simulink model "cart_model"  (R2015b)
settings: Solver=VariableStepAuto  StartTime=0.0  StopTime=20  RelTol=1e-3
InitFcn:
  | [g,m1,T1,f_1s,f_1k,m2,l,f_2k,M_sp,f_1k_lin,f_2k_lin,k1,k2] =...
  |     set_system_parameters()
values from neighbouring files (symbols this model uses):
  f_1k = f_1s * 0.9    (= 0.143348623853)    [set_system_parameters.m]
  f_1k_lin = 8    [set_system_parameters.m]
  f_1s = T1 / (m1 * g)    (= 0.159276248726)    [set_system_parameters.m]
  f_2k = 0.0062586    [set_system_parameters.m]
  f_2k_lin = 0.01    [set_system_parameters.m]
  g = 9.81    [set_system_parameters.m]
  k1 = -200    [set_system_parameters.m]
  k2 = -5    [set_system_parameters.m]
  l = 2/3 * l_physical    (= 0.466666666667)    [set_system_parameters.m]
  m1 = 1.6    [set_system_parameters.m]
  m2 = 55/1000    (= 0.055)    [set_system_parameters.m]
  M_sp = 0.0065    [set_system_parameters.m]
undefined symbols (not defined in the file or in its folder): sgn, zh_step
libraries: simulink x2
settings Model: Creator=Anony  LastModifiedBy=Anony

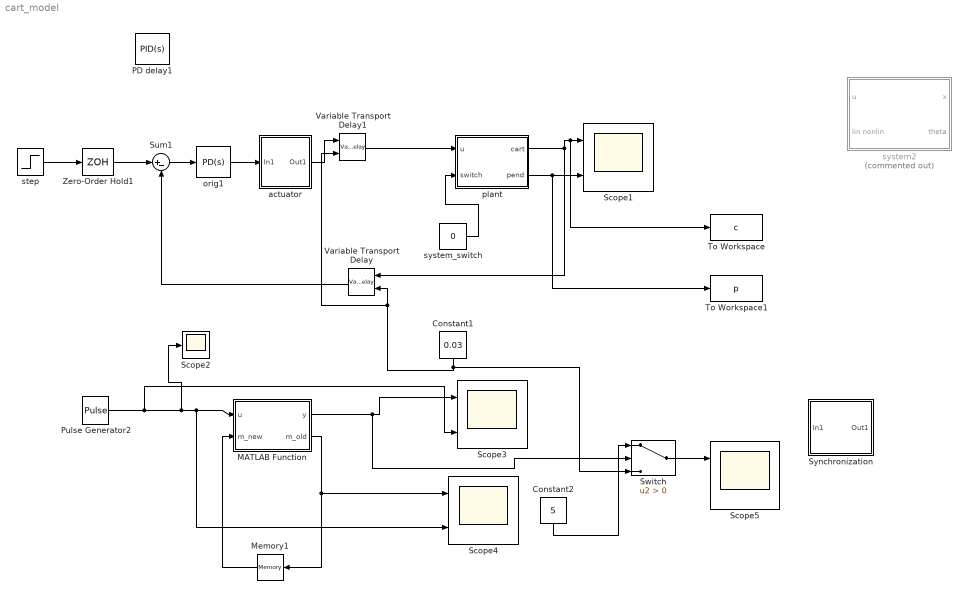
== system cart_model ==
  Constant1 : Constant  Value=0.03
  Constant2 : Constant  Value=5
  MATLAB Function : MATLAB Function  TreatAsAtomicUnit=on
  Memory1 : Memory
  PD delay1 : simulink/Continuous/PID Controller  Controller=PID  TimeDomain=Continuous-time  SampleTime=-1  IntegratorMethod=Forward Euler  FilterMethod=Forward Euler  Form=Parallel  UseFilter=on  ControllerParametersSource=internal  P=44.2780709689467  I=5.84490047291559  D=15.97815467959  N=2.77235262395788  InitialConditionSource=internal  InitialConditionForIntegrator=0  InitialConditionForFilter=0  ExternalReset=none  LimitOutput=on  UpperSaturationLimit=5/1000  LowerSaturationLimit=-5/1000  LinearizeAsGain=on  AntiWindupMode=none  Kb=1  TrackingMode=off  Kt=1  PParamMin=[]  PParamMax=[]  IParamMin=[]  IParamMax=[]  DParamMin=[]  DParamMax=[]  NParamMin=[]  NParamMax=[]  KbParamMin=[]  KbParamMax=[]  KtParamMin=[]  KtParamMax=[]  POutMin=[]  POutMax=[]  IOutMin=[]  IOutMax=[]  DOutMin=[]  DOutMax=[]  NOutMin=[]  NOutMax=[]  KbOutMin=[]  KbOutMax=[]  KtOutMin=[]  KtOutMax=[]  IntegratorOutMin=[]  IntegratorOutMax=[]  FilterOutMin=[]  FilterOutMax=[]  SumOutMin=[]  SumOutMax=[]  SumI1OutMin=[]  SumI1OutMax=[]  SumI2OutMin=[]  SumI2OutMax=[]  SumI3OutMin=[]  SumI3OutMax=[]  SumDOutMin=[]  SumDOutMax=[]  SaturationOutMin=[]  SaturationOutMax=[]  IntegratorContinuousStateAttributes=''  IntegratorStateMustResolveToSignalObject=off  IntegratorRTWStateStorageClass=Auto  FilterContinuousStateAttributes=''  FilterStateMustResolveToSignalObject=off  FilterRTWStateStorageClass=Auto  DifferentiatorICPrevScaledInput=0  DifferentiatorOutMin=[]  DifferentiatorOutMax=[]
  Pulse Generator2 : DiscretePulseGenerator  PulseType=Time based  Period=0.1
  Scope{1,3..5} (4 alike) : Scope  NumInputPorts=2
  Scope2 : Scope
  Sum1 : Sum  Inputs=|+-
  Switch : Switch  Criteria=u2 > Threshold
  Synchronization : Subsystem
  To Workspace : ToWorkspace  VariableName=c  SaveFormat=Timeseries  SampleTime=-1
  To Workspace1 : ToWorkspace  VariableName=p  SaveFormat=Timeseries  SampleTime=-1
  Variable Transport Delay : VariableTransportDelay  VariableDelayType=Variable transport delay  MaximumDelay=10
  Variable Transport Delay1 : VariableTransportDelay  VariableDelayType=Variable transport delay  MaximumDelay=10
  Zero-Order Hold1 : ZeroOrderHold  SampleTime=0.01
  actuator : Subsystem
  orig1 : simulink/Continuous/PID Controller  Controller=PD  TimeDomain=Continuous-time  SampleTime=-1  IntegratorMethod=Forward Euler  FilterMethod=Forward Euler  Form=Parallel  UseFilter=on  ControllerParametersSource=internal  P=0.0142  I=0.0175856984919557  D=0.0001  N=100  InitialConditionSource=internal  InitialConditionForIntegrator=0  InitialConditionForFilter=0  ExternalReset=none  LimitOutput=on  UpperSaturationLimit=5/1000  LowerSaturationLimit=-5/1000  LinearizeAsGain=on  AntiWindupMode=none  Kb=1  TrackingMode=off  Kt=1  PParamMin=[]  PParamMax=[]  IParamMin=[]  IParamMax=[]  DParamMin=[]  DParamMax=[]  NParamMin=[]  NParamMax=[]  KbParamMin=[]  KbParamMax=[]  KtParamMin=[]  KtParamMax=[]  POutMin=[]  POutMax=[]  IOutMin=[]  IOutMax=[]  DOutMin=[]  DOutMax=[]  NOutMin=[]  NOutMax=[]  KbOutMin=[]  KbOutMax=[]  KtOutMin=[]  KtOutMax=[]  IntegratorOutMin=[]  IntegratorOutMax=[]  FilterOutMin=[]  FilterOutMax=[]  SumOutMin=[]  SumOutMax=[]  SumI1OutMin=[]  SumI1OutMax=[]  SumI2OutMin=[]  SumI2OutMax=[]  SumI3OutMin=[]  SumI3OutMax=[]  SumDOutMin=[]  SumDOutMax=[]  SaturationOutMin=[]  SaturationOutMax=[]  IntegratorContinuousStateAttributes=''  IntegratorStateMustResolveToSignalObject=off  IntegratorRTWStateStorageClass=Auto  FilterContinuousStateAttributes=''  FilterStateMustResolveToSignalObject=off  FilterRTWStateStorageClass=Auto  DifferentiatorICPrevScaledInput=0  DifferentiatorOutMin=[]  DifferentiatorOutMax=[]
  plant : Subsystem
  step : Step  After=0.15  SampleTime=0
  system2 : Subsystem  Commented=on
  system_switch : Constant  Value=0
  wires:
  plant/2(pend) -> To Workspace1/1, Scope1/2
  orig1/1 -> actuator/1(In1)
  Sum1/1 -> orig1/1
  Zero-Order Hold1/1 -> Sum1/1
  actuator/1(Out1) -> Variable Transport Delay1/1
  plant/1(cart) -> Variable Transport Delay/1, To Workspace/1, Scope1/1
  Constant1/1 -> Switch/3, Variable Transport Delay1/2, Variable Transport Delay/2
  system_switch/1 -> plant/2(switch)
  step/1 -> Zero-Order Hold1/1
  Variable Transport Delay1/1 -> plant/1(u)
  Variable Transport Delay/1 -> Sum1/2
  MATLAB Function/2(m_old) -> Memory1/1, Scope4/1
  Memory1/1 -> MATLAB Function/2(m_new)
  MATLAB Function/1(y) -> Switch/2, Scope3/1
  Pulse Generator2/1 -> Scope3/2, Scope2/1, Scope4/2, MATLAB Function/1(u)
  Constant2/1 -> Switch/1
  Switch/1 -> Scope5/1

== system cart_model/Synchronization ==
  In1 : Inport
  MATLAB Function1 : MATLAB Function  TreatAsAtomicUnit=on
  Memory2 : Memory
  Out1 : Outport
  wires:
  MATLAB Function1/2(m_old) -> Memory2/1
  Memory2/1 -> MATLAB Function1/2(m_new)
  In1/1 -> MATLAB Function1/1(u)
  MATLAB Function1/1(y) -> Out1/1

== system cart_model/actuator ==
  In1 : Inport
  V > N1 : Gain  Gain=4
  mv > V1 : Gain  Gain=1000
  Out1 : Outport
  wires:
  V > N1/1 -> Out1/1
  mv > V1/1 -> V > N1/1
  In1/1 -> mv > V1/1

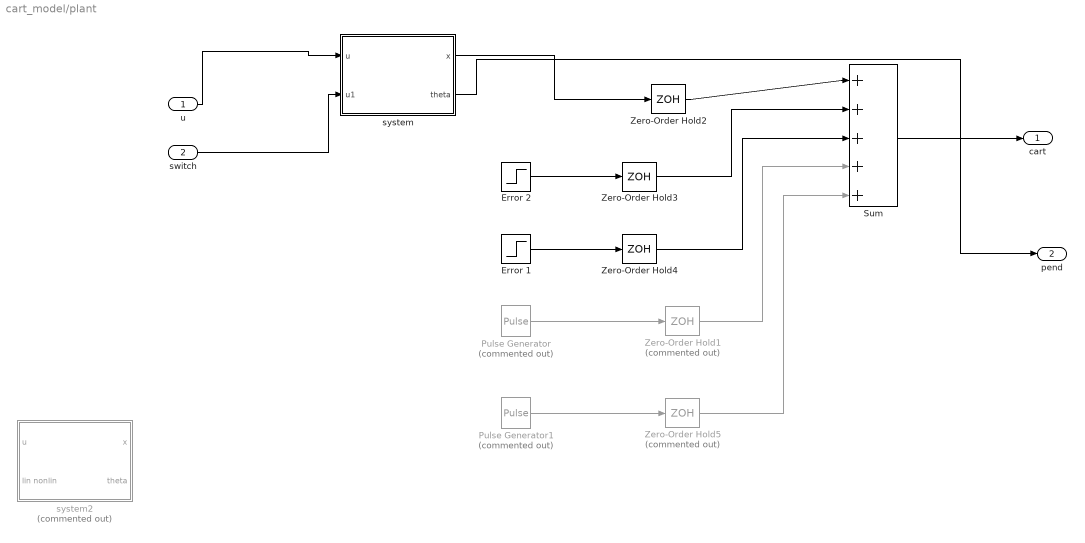
== system cart_model/plant ==
  u : Inport
  switch : Inport  Port=2
  Error 1 : Step  Time=15  After=0.02  SampleTime=0
  Error 2 : Step  Time=10  After=-0.02  SampleTime=0
  Pulse Generator : DiscretePulseGenerator  Commented=on  PulseType=Time based  Amplitude=0.3  Period=3  PulseWidth=5  PhaseDelay=15
  Pulse Generator1 : DiscretePulseGenerator  Commented=on  PulseType=Time based  Amplitude=-0.18  Period=3  PulseWidth=5  PhaseDelay=25
  Sum : Sum  Inputs=|+++++
  Zero-Order Hold1 : ZeroOrderHold  Commented=on  SampleTime=zh_step
  Zero-Order Hold2 : ZeroOrderHold  SampleTime=zh_step
  Zero-Order Hold3 : ZeroOrderHold  SampleTime=zh_step
  Zero-Order Hold4 : ZeroOrderHold  SampleTime=zh_step
  Zero-Order Hold5 : ZeroOrderHold  Commented=on  SampleTime=zh_step
  system : Subsystem
  system2 : Subsystem  Commented=on
  cart : Outport
  pend : Outport  Port=2
  wires:
  system/2(theta) -> pend/1
  switch/1 -> system/2(u1)
  u/1 -> system/1(u)
  Zero-Order Hold5/1 -> Sum/5
  Pulse Generator1/1 -> Zero-Order Hold5/1
  Zero-Order Hold1/1 -> Sum/4
  Pulse Generator/1 -> Zero-Order Hold1/1
  Error 1/1 -> Zero-Order Hold4/1
  system/1(x) -> Zero-Order Hold2/1
  Error 2/1 -> Zero-Order Hold3/1
  Sum/1 -> cart/1
  Zero-Order Hold2/1 -> Sum/1
  Zero-Order Hold3/1 -> Sum/2
  Zero-Order Hold4/1 -> Sum/3

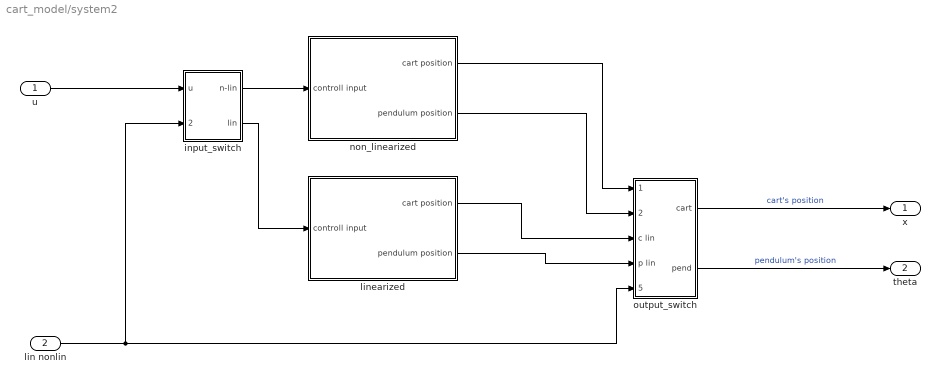
== system cart_model/system2 ==
  u : Inport
  lin nonlin : Inport  Port=2
  input_switch : Subsystem
  linearized : Subsystem
  non_linearized : Subsystem
  output_switch : Subsystem
  x : Outport
  theta : Outport  Port=2
  wires:
  lin nonlin/1 -> input_switch/2(switch), output_switch/5(switch)
  u/1 -> input_switch/1(u)
  output_switch/2(pend) -> theta/1  "pendulum's position"
  linearized/2("pendulum position ") -> output_switch/4(p lin)
  linearized/1(cart position) -> output_switch/3(c lin)
  non_linearized/2("pendulum position ") -> output_switch/2(p n-lin)
  non_linearized/1(cart position) -> output_switch/1(c n-lin)
  output_switch/1(cart) -> x/1  "cart's position"
  input_switch/2("lin ") -> linearized/1(controll input)
  input_switch/1(n-lin) -> non_linearized/1(controll input)

== system cart_model/plant/system ==
  u : Inport
  u1 : Inport  Port=2
  input_switch : Subsystem
  linearized : Subsystem
  non_linearized : Subsystem
  output_switch : Subsystem
  x : Outport
  theta : Outport  Port=2
  wires:
  u1/1 -> input_switch/2(switch), output_switch/5(switch)
  u/1 -> input_switch/1(u)
  output_switch/2(pend) -> theta/1  "pendulum's position"
  linearized/2("pendulum position ") -> output_switch/4(p lin)
  linearized/1(cart position) -> output_switch/3(c lin)
  non_linearized/2("pendulum position ") -> output_switch/2(p n-lin)
  non_linearized/1(cart position) -> output_switch/1(c n-lin)
  output_switch/1(cart) -> x/1  "cart's position"
  input_switch/2("lin ") -> linearized/1(controll input)
  input_switch/1(n-lin) -> non_linearized/1(controll input)

== system cart_model/plant/system2 ==
  u : Inport
  lin nonlin : Inport  Port=2
  input_switch : Subsystem
  linearized : Subsystem
  non_linearized : Subsystem
  output_switch : Subsystem
  x : Outport
  theta : Outport  Port=2
  wires:
  input_switch/1(n-lin) -> non_linearized/1(controll input)
  input_switch/2("lin ") -> linearized/1(controll input)
  output_switch/1(cart) -> x/1  "cart's position"
  non_linearized/1(cart position) -> output_switch/1(c n-lin)
  non_linearized/2("pendulum position ") -> output_switch/2(p n-lin)
  linearized/1(cart position) -> output_switch/3(c lin)
  linearized/2("pendulum position ") -> output_switch/4(p lin)
  output_switch/2(pend) -> theta/1  "pendulum's position"
  u/1 -> input_switch/1(u)
  lin nonlin/1 -> output_switch/5(switch), input_switch/2(switch)

== system cart_model/system2/input_switch ==
  u : Inport
  switch : Inport  Port=2
  Switch2 : Switch  Criteria=u2 ~= 0  Threshold=1
  Switch3 : Switch  Criteria=u2 ~= 0  Threshold=1
  n-lin : Outport
  "lin " : Outport  Port=2
  wires:
  switch/1 -> Switch3/2, Switch2/2
  u/1 -> Switch3/1, Switch2/3
  Switch2/1 -> "lin "/1
  Switch3/1 -> n-lin/1

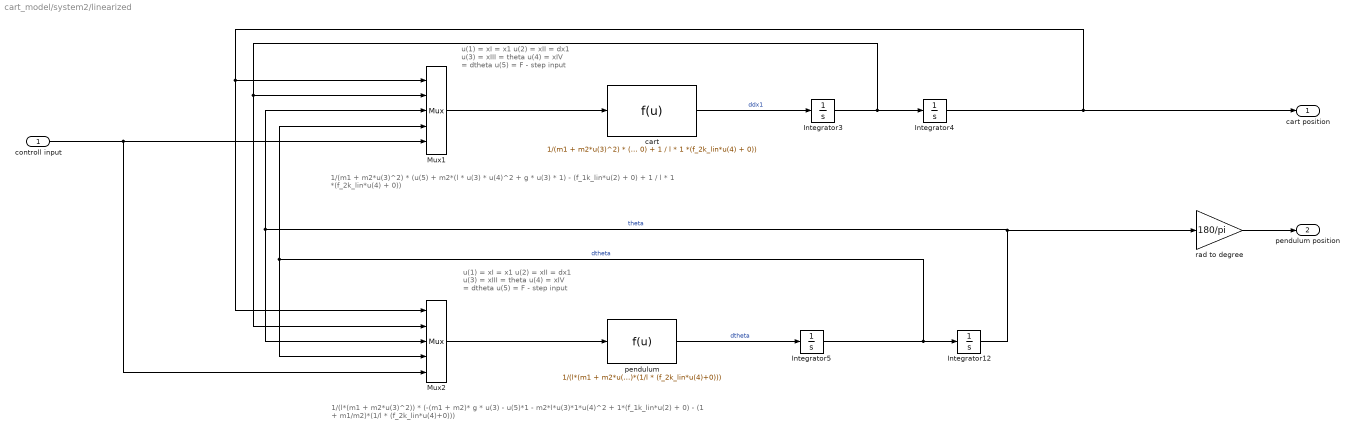
== system cart_model/system2/linearized ==
  note: 1/(l*(m1 + m2*u(3)^2)) * (-(m1 + m2)* g * u(3) - u(5)*1 - m2*l*u(3)*1*u(4)^2 + 1*(f_1k_lin*u(2) + 0) - (1 + m1/m2)*(1/l * (f_2k_lin*u(4)+0)))
  note: 1/(m1 + m2*u(3)^2) * (u(5) + m2*(l * u(3) * u(4)^2 + g * u(3) * 1) - (f_1k_lin*u(2) + 0) + 1 / l * 1 *(f_2k_lin*u(4) + 0))
  note: u(1) = xI = x1
      | u(2) = xII = dx1
      | u(3) = xIII = theta
      | u(4) = xIV = dtheta
      | u(5) = F - step input
  note: u(1) = xI = x1
      | u(2) = xII = dx1
      | u(3) = xIII = theta
      | u(4) = xIV = dtheta
      | u(5) = F - step input
  controll input : Inport
  Integrator{3..5,12} (4 alike) : Integrator
  Mux1 : Mux  Inputs=5
  Mux2 : Mux  Inputs=5
  cart : Fcn  Expr=1/(m1 + m2*u(3)^2) * (u(5) + m2*(l * u(3) * u(4)^2 + g * u(3) * 1) - (f_1k_lin*u(2) + 0) + 1 / l * 1 *(f_2k_lin*u(4) + 0))
  "pendulum " : Fcn  Expr=1/(l*(m1 + m2*u(3)^2)) * (-(m1 + m2)* g * u(3) - u(5)*1 - m2*l*u(3)*1*u(4)^2 + 1*(f_1k_lin*u(2) + 0) - (1 + m1/m2)*(1/l * (f_2k_lin*u(4)+0)))
  rad to degree : Gain  Gain=180/pi
  cart position : Outport
  "pendulum position " : Outport  Port=2
  wires:
  controll input/1 -> Mux1/5, Mux2/5
  Integrator4/1 -> cart position/1, Mux2/1, Mux1/1
  Integrator3/1 -> Integrator4/1, Mux2/2, Mux1/2
  cart/1 -> Integrator3/1  "ddx1"
  Mux2/1 -> "pendulum "/1
  "pendulum "/1 -> Integrator5/1  "dtheta"
  Integrator5/1 -> Integrator12/1, Mux1/4, Mux2/4  "dtheta"
  Integrator12/1 -> rad to degree/1, Mux1/3, Mux2/3  "theta"
  Mux1/1 -> cart/1
  rad to degree/1 -> "pendulum position "/1

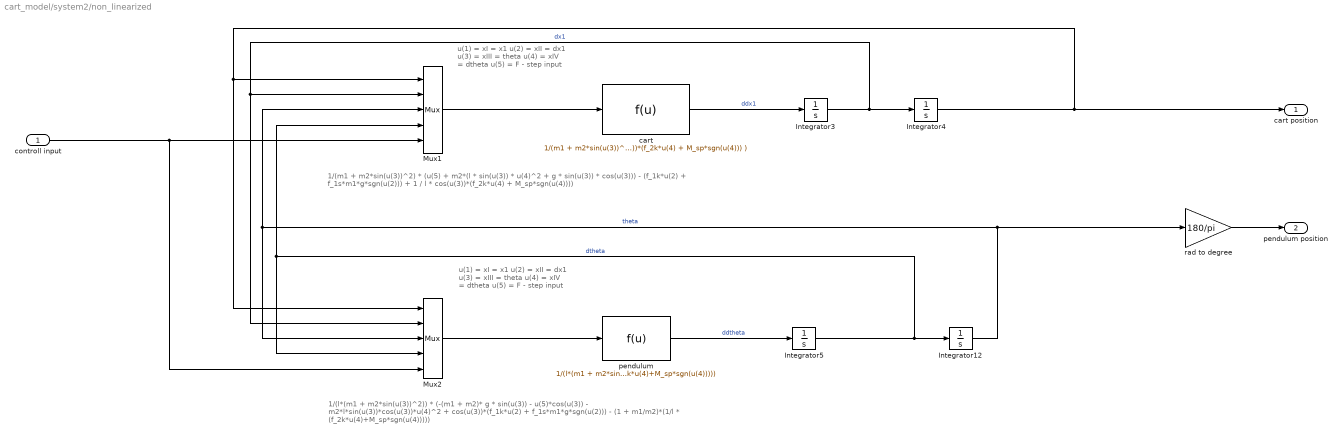
== system cart_model/system2/non_linearized ==
  note: u(1) = xI = x1
      | u(2) = xII = dx1
      | u(3) = xIII = theta
      | u(4) = xIV = dtheta
      | u(5) = F - step input
  note: u(1) = xI = x1
      | u(2) = xII = dx1
      | u(3) = xIII = theta
      | u(4) = xIV = dtheta
      | u(5) = F - step input
  note: 1/(m1 + m2*sin(u(3))^2) * (u(5) + m2*(l * sin(u(3)) * u(4)^2 + g * sin(u(3)) * cos(u(3))) - (f_1k*u(2) + f_1s*m1*g*sgn(u(2))) + 1 / l * cos(u(3))*(f_2k*u(4) + M_sp*sgn(u(4))))
  note: 1/(l*(m1 + m2*sin(u(3))^2)) * (-(m1 + m2)* g * sin(u(3)) - u(5)*cos(u(3)) - m2*l*sin(u(3))*cos(u(3))*u(4)^2 + cos(u(3))*(f_1k*u(2) + f_1s*m1*g*sgn(u(2))) - (1 + m1/m2)*(1/l * (f_2k*u(4)+M_sp*sgn(u(4)))))
  controll input : Inport
  Integrator{3..5,12} (4 alike) : Integrator
  Mux1 : Mux  Inputs=5
  Mux2 : Mux  Inputs=5
  cart : Fcn  Expr=1/(m1 + m2*sin(u(3))^2) * (u(5) + m2*(l * sin(u(3)) * u(4)^2 + g * sin(u(3)) * cos(u(3))) - (f_1k*u(2) + f_1s*m1*g*sgn(u(2))) + 1 / l * cos(u(3))*(f_2k*u(4) + M_sp*sgn(u(4))) )
  "pendulum " : Fcn  Expr=1/(l*(m1 + m2*sin(u(3))^2)) * (-(m1 + m2)* g * sin(u(3)) - u(5)*cos(u(3)) - m2*l*sin(u(3))*cos(u(3))*u(4)^2 + cos(u(3))*(f_1k*u(2) + f_1s*m1*g*sgn(u(2))) - (1 + m1/m2)*(1/l * (f_2k*u(4)+M_sp*sgn(u(4)))))
  rad to degree : Gain  Gain=180/pi
  cart position : Outport
  "pendulum position " : Outport  Port=2
  wires:
  controll input/1 -> Mux1/5, Mux2/5
  Integrator4/1 -> Mux1/1, Mux2/1, cart position/1
  rad to degree/1 -> "pendulum position "/1
  Mux1/1 -> cart/1
  Integrator12/1 -> Mux2/3, Mux1/3, rad to degree/1  "theta"
  Integrator3/1 -> Mux1/2, Mux2/2, Integrator4/1  "dx1"
  Integrator5/1 -> Mux2/4, Mux1/4, Integrator12/1  "dtheta"
  "pendulum "/1 -> Integrator5/1  "ddtheta"
  Mux2/1 -> "pendulum "/1
  cart/1 -> Integrator3/1  "ddx1"

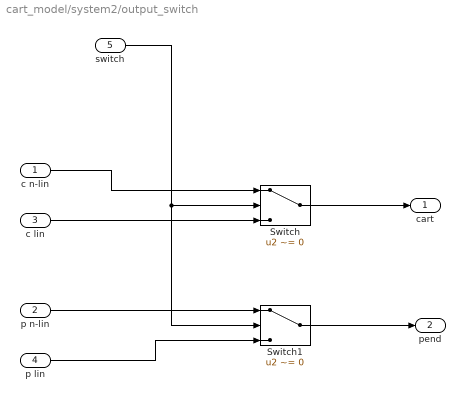
== system cart_model/system2/output_switch ==
  c n-lin : Inport
  p n-lin : Inport  Port=2
  c lin : Inport  Port=3
  p lin : Inport  Port=4
  switch : Inport  Port=5
  Switch : Switch  Criteria=u2 ~= 0  Threshold=1
  Switch1 : Switch  Criteria=u2 ~= 0  Threshold=1
  cart : Outport
  pend : Outport  Port=2
  wires:
  p n-lin/1 -> Switch1/1
  c n-lin/1 -> Switch/1
  Switch1/1 -> pend/1
  c lin/1 -> Switch/3
  Switch/1 -> cart/1
  p lin/1 -> Switch1/3
  switch/1 -> Switch/2, Switch1/2

== system cart_model/plant/system/input_switch ==
  u : Inport
  switch : Inport  Port=2
  Switch2 : Switch  Criteria=u2 ~= 0  Threshold=1
  Switch3 : Switch  Criteria=u2 ~= 0  Threshold=1
  c : Constant  Value=0
  n-lin : Outport
  "lin " : Outport  Port=2
  wires:
  switch/1 -> Switch3/2, Switch2/2
  u/1 -> Switch3/1, Switch2/3
  Switch2/1 -> "lin "/1
  Switch3/1 -> n-lin/1
  c/1 -> Switch2/1, Switch3/3

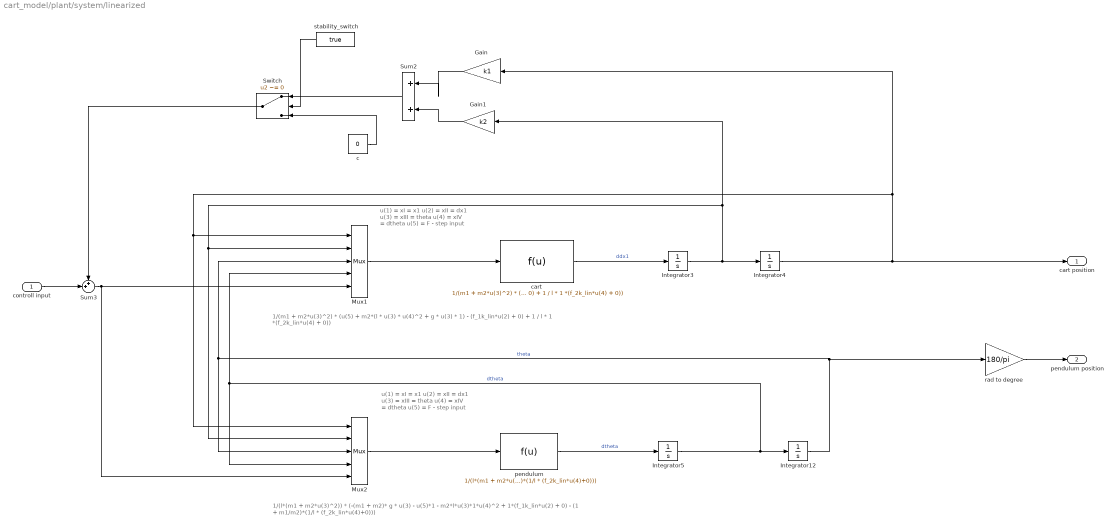
== system cart_model/plant/system/linearized ==
  note: 1/(l*(m1 + m2*u(3)^2)) * (-(m1 + m2)* g * u(3) - u(5)*1 - m2*l*u(3)*1*u(4)^2 + 1*(f_1k_lin*u(2) + 0) - (1 + m1/m2)*(1/l * (f_2k_lin*u(4)+0)))
  note: 1/(m1 + m2*u(3)^2) * (u(5) + m2*(l * u(3) * u(4)^2 + g * u(3) * 1) - (f_1k_lin*u(2) + 0) + 1 / l * 1 *(f_2k_lin*u(4) + 0))
  note: u(1) = xI = x1
      | u(2) = xII = dx1
      | u(3) = xIII = theta
      | u(4) = xIV = dtheta
      | u(5) = F - step input
  note: u(1) = xI = x1
      | u(2) = xII = dx1
      | u(3) = xIII = theta
      | u(4) = xIV = dtheta
      | u(5) = F - step input
  controll input : Inport
  Gain : Gain  Gain=k1
  Gain1 : Gain  Gain=k2
  Integrator{3..5,12} (4 alike) : Integrator
  Mux1 : Mux  Inputs=5
  Mux2 : Mux  Inputs=5
  Sum2 : Sum  Inputs=|++
  Sum3 : Sum  Inputs=++|
  Switch : Switch  Criteria=u2 ~= 0
  c : Constant  Value=0
  cart : Fcn  Expr=1/(m1 + m2*u(3)^2) * (u(5) + m2*(l * u(3) * u(4)^2 + g * u(3) * 1) - (f_1k_lin*u(2) + 0) + 1 / l * 1 *(f_2k_lin*u(4) + 0))
  "pendulum " : Fcn  Expr=1/(l*(m1 + m2*u(3)^2)) * (-(m1 + m2)* g * u(3) - u(5)*1 - m2*l*u(3)*1*u(4)^2 + 1*(f_1k_lin*u(2) + 0) - (1 + m1/m2)*(1/l * (f_2k_lin*u(4)+0)))
  rad to degree : Gain  Gain=180/pi
  stability_switch : Constant  Value=true
  cart position : Outport
  "pendulum position " : Outport  Port=2
  wires:
  stability_switch/1 -> Switch/2
  Switch/1 -> Sum3/1
  Sum2/1 -> Switch/1
  Sum3/1 -> Mux1/5, Mux2/5
  controll input/1 -> Sum3/2
  Gain1/1 -> Sum2/2
  Gain/1 -> Sum2/1
  Integrator4/1 -> cart position/1, Mux2/1, Mux1/1, Gain/1
  Integrator3/1 -> Integrator4/1, Mux2/2, Mux1/2, Gain1/1
  cart/1 -> Integrator3/1  "ddx1"
  Mux2/1 -> "pendulum "/1
  "pendulum "/1 -> Integrator5/1  "dtheta"
  Integrator5/1 -> Integrator12/1, Mux1/4, Mux2/4  "dtheta"
  Integrator12/1 -> rad to degree/1, Mux1/3, Mux2/3  "theta"
  Mux1/1 -> cart/1
  rad to degree/1 -> "pendulum position "/1
  c/1 -> Switch/3

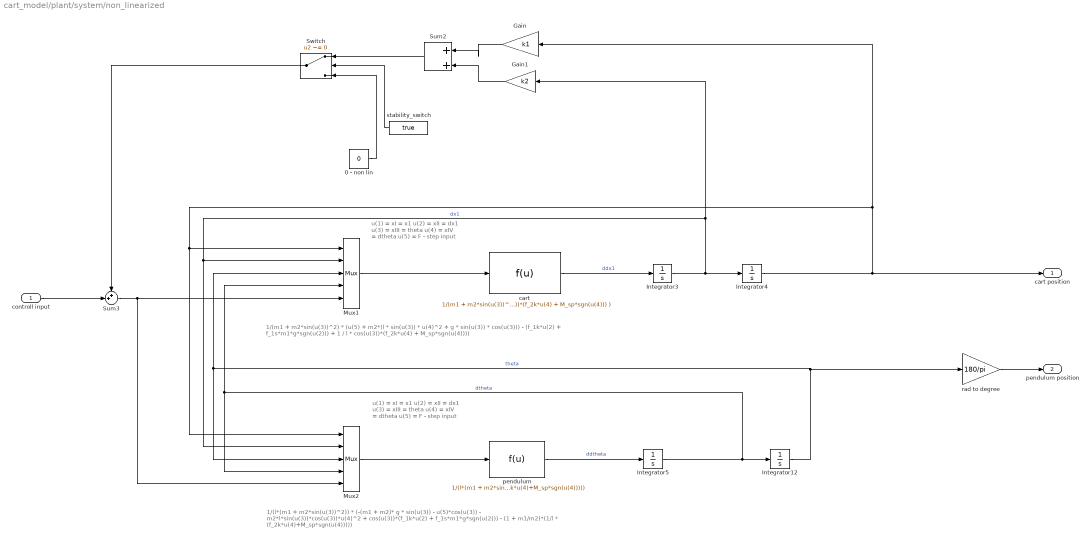
== system cart_model/plant/system/non_linearized ==
  note: u(1) = xI = x1
      | u(2) = xII = dx1
      | u(3) = xIII = theta
      | u(4) = xIV = dtheta
      | u(5) = F - step input
  note: u(1) = xI = x1
      | u(2) = xII = dx1
      | u(3) = xIII = theta
      | u(4) = xIV = dtheta
      | u(5) = F - step input
  note: 1/(m1 + m2*sin(u(3))^2) * (u(5) + m2*(l * sin(u(3)) * u(4)^2 + g * sin(u(3)) * cos(u(3))) - (f_1k*u(2) + f_1s*m1*g*sgn(u(2))) + 1 / l * cos(u(3))*(f_2k*u(4) + M_sp*sgn(u(4))))
  note: 1/(l*(m1 + m2*sin(u(3))^2)) * (-(m1 + m2)* g * sin(u(3)) - u(5)*cos(u(3)) - m2*l*sin(u(3))*cos(u(3))*u(4)^2 + cos(u(3))*(f_1k*u(2) + f_1s*m1*g*sgn(u(2))) - (1 + m1/m2)*(1/l * (f_2k*u(4)+M_sp*sgn(u(4)))))
  controll input : Inport
  0 - non lin : Constant  Value=0
  Gain : Gain  Gain=k1
  Gain1 : Gain  Gain=k2
  Integrator{3..5,12} (4 alike) : Integrator
  Mux1 : Mux  Inputs=5
  Mux2 : Mux  Inputs=5
  Sum2 : Sum  Inputs=|++
  Sum3 : Sum  Inputs=++|
  Switch : Switch  Criteria=u2 ~= 0
  cart : Fcn  Expr=1/(m1 + m2*sin(u(3))^2) * (u(5) + m2*(l * sin(u(3)) * u(4)^2 + g * sin(u(3)) * cos(u(3))) - (f_1k*u(2) + f_1s*m1*g*sgn(u(2))) + 1 / l * cos(u(3))*(f_2k*u(4) + M_sp*sgn(u(4))) )
  "pendulum " : Fcn  Expr=1/(l*(m1 + m2*sin(u(3))^2)) * (-(m1 + m2)* g * sin(u(3)) - u(5)*cos(u(3)) - m2*l*sin(u(3))*cos(u(3))*u(4)^2 + cos(u(3))*(f_1k*u(2) + f_1s*m1*g*sgn(u(2))) - (1 + m1/m2)*(1/l * (f_2k*u(4)+M_sp*sgn(u(4)))))
  rad to degree : Gain  Gain=180/pi
  stability_switch : Constant  Value=true
  cart position : Outport
  "pendulum position " : Outport  Port=2
  wires:
  Sum3/1 -> Mux1/5, Mux2/5
  controll input/1 -> Sum3/2
  stability_switch/1 -> Switch/2
  Switch/1 -> Sum3/1
  Sum2/1 -> Switch/1
  Gain1/1 -> Sum2/2
  Gain/1 -> Sum2/1
  Integrator4/1 -> Mux1/1, Mux2/1, Gain/1, cart position/1
  rad to degree/1 -> "pendulum position "/1
  Mux1/1 -> cart/1
  Integrator12/1 -> Mux2/3, Mux1/3, rad to degree/1  "theta"
  Integrator3/1 -> Mux1/2, Mux2/2, Gain1/1, Integrator4/1  "dx1"
  Integrator5/1 -> Mux2/4, Mux1/4, Integrator12/1  "dtheta"
  "pendulum "/1 -> Integrator5/1  "ddtheta"
  Mux2/1 -> "pendulum "/1
  cart/1 -> Integrator3/1  "ddx1"
  0 - non lin/1 -> Switch/3

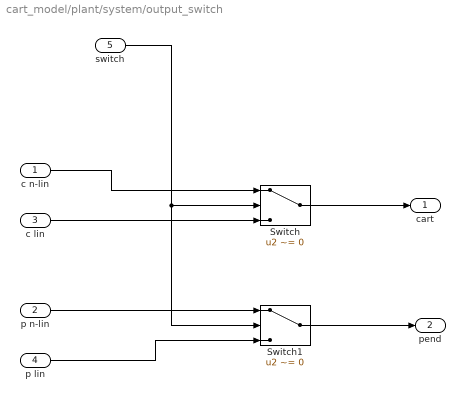
== system cart_model/plant/system/output_switch ==
  c n-lin : Inport
  p n-lin : Inport  Port=2
  c lin : Inport  Port=3
  p lin : Inport  Port=4
  switch : Inport  Port=5
  Switch : Switch  Criteria=u2 ~= 0  Threshold=1
  Switch1 : Switch  Criteria=u2 ~= 0  Threshold=1
  cart : Outport
  pend : Outport  Port=2
  wires:
  p n-lin/1 -> Switch1/1
  c n-lin/1 -> Switch/1
  Switch1/1 -> pend/1
  c lin/1 -> Switch/3
  Switch/1 -> cart/1
  p lin/1 -> Switch1/3
  switch/1 -> Switch/2, Switch1/2

== system cart_model/plant/system2/input_switch ==
  u : Inport
  switch : Inport  Port=2
  Constant : Constant  Value=0
  Switch2 : Switch  Criteria=u2 ~= 0  Threshold=1
  Switch3 : Switch  Criteria=u2 ~= 0  Threshold=1
  n-lin : Outport
  "lin " : Outport  Port=2
  wires:
  Switch3/1 -> n-lin/1
  Switch2/1 -> "lin "/1
  u/1 -> Switch2/3, Switch3/1
  switch/1 -> Switch2/2, Switch3/2
  Constant/1 -> Switch2/1, Switch3/3

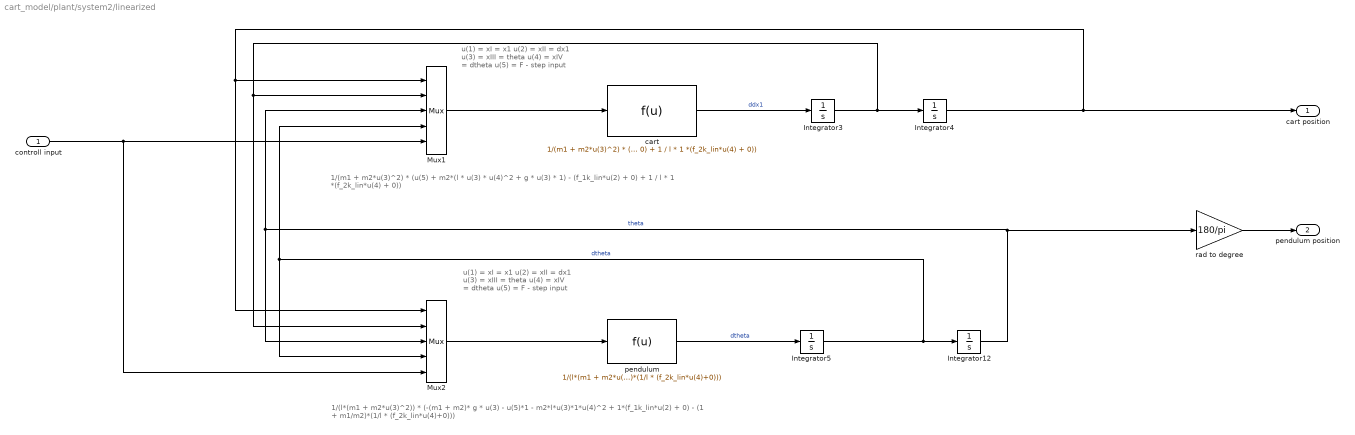
== system cart_model/plant/system2/linearized ==
  note: u(1) = xI = x1
      | u(2) = xII = dx1
      | u(3) = xIII = theta
      | u(4) = xIV = dtheta
      | u(5) = F - step input
  note: u(1) = xI = x1
      | u(2) = xII = dx1
      | u(3) = xIII = theta
      | u(4) = xIV = dtheta
      | u(5) = F - step input
  note: 1/(m1 + m2*u(3)^2) * (u(5) + m2*(l * u(3) * u(4)^2 + g * u(3) * 1) - (f_1k_lin*u(2) + 0) + 1 / l * 1 *(f_2k_lin*u(4) + 0))
  note: 1/(l*(m1 + m2*u(3)^2)) * (-(m1 + m2)* g * u(3) - u(5)*1 - m2*l*u(3)*1*u(4)^2 + 1*(f_1k_lin*u(2) + 0) - (1 + m1/m2)*(1/l * (f_2k_lin*u(4)+0)))
  controll input : Inport
  Integrator{3..5,12} (4 alike) : Integrator
  Mux1 : Mux  Inputs=5
  Mux2 : Mux  Inputs=5
  cart : Fcn  Expr=1/(m1 + m2*u(3)^2) * (u(5) + m2*(l * u(3) * u(4)^2 + g * u(3) * 1) - (f_1k_lin*u(2) + 0) + 1 / l * 1 *(f_2k_lin*u(4) + 0))
  "pendulum " : Fcn  Expr=1/(l*(m1 + m2*u(3)^2)) * (-(m1 + m2)* g * u(3) - u(5)*1 - m2*l*u(3)*1*u(4)^2 + 1*(f_1k_lin*u(2) + 0) - (1 + m1/m2)*(1/l * (f_2k_lin*u(4)+0)))
  rad to degree : Gain  Gain=180/pi
  cart position : Outport
  "pendulum position " : Outport  Port=2
  wires:
  rad to degree/1 -> "pendulum position "/1
  Mux1/1 -> cart/1
  Integrator12/1 -> Mux2/3, Mux1/3, rad to degree/1  "theta"
  Integrator5/1 -> Mux2/4, Mux1/4, Integrator12/1  "dtheta"
  "pendulum "/1 -> Integrator5/1  "dtheta"
  Mux2/1 -> "pendulum "/1
  cart/1 -> Integrator3/1  "ddx1"
  Integrator3/1 -> Mux1/2, Mux2/2, Integrator4/1
  Integrator4/1 -> Mux1/1, Mux2/1, cart position/1
  controll input/1 -> Mux2/5, Mux1/5

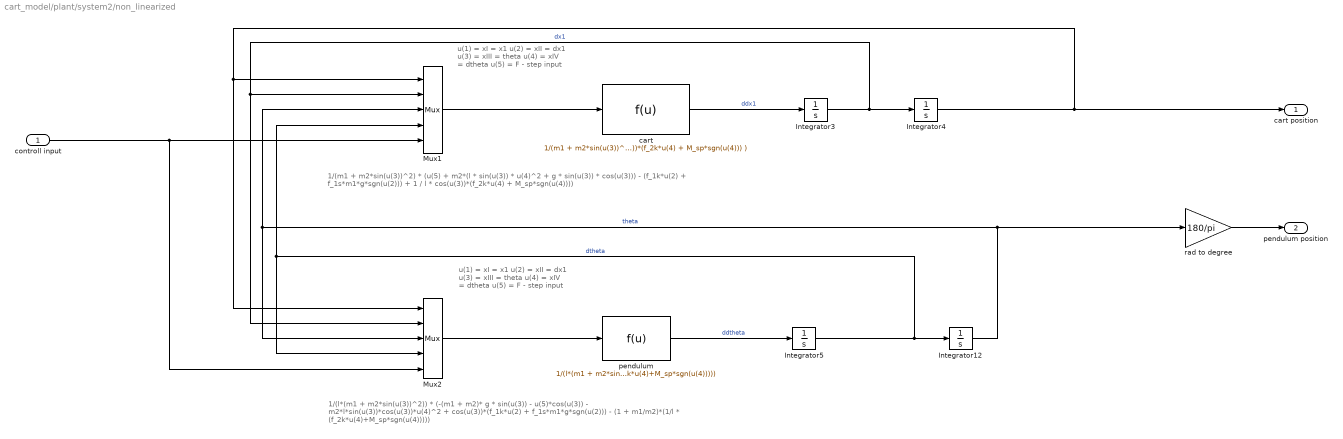
== system cart_model/plant/system2/non_linearized ==
  note: 1/(l*(m1 + m2*sin(u(3))^2)) * (-(m1 + m2)* g * sin(u(3)) - u(5)*cos(u(3)) - m2*l*sin(u(3))*cos(u(3))*u(4)^2 + cos(u(3))*(f_1k*u(2) + f_1s*m1*g*sgn(u(2))) - (1 + m1/m2)*(1/l * (f_2k*u(4)+M_sp*sgn(u(4)))))
  note: 1/(m1 + m2*sin(u(3))^2) * (u(5) + m2*(l * sin(u(3)) * u(4)^2 + g * sin(u(3)) * cos(u(3))) - (f_1k*u(2) + f_1s*m1*g*sgn(u(2))) + 1 / l * cos(u(3))*(f_2k*u(4) + M_sp*sgn(u(4))))
  note: u(1) = xI = x1
      | u(2) = xII = dx1
      | u(3) = xIII = theta
      | u(4) = xIV = dtheta
      | u(5) = F - step input
  note: u(1) = xI = x1
      | u(2) = xII = dx1
      | u(3) = xIII = theta
      | u(4) = xIV = dtheta
      | u(5) = F - step input
  controll input : Inport
  Integrator{3..5,12} (4 alike) : Integrator
  Mux1 : Mux  Inputs=5
  Mux2 : Mux  Inputs=5
  cart : Fcn  Expr=1/(m1 + m2*sin(u(3))^2) * (u(5) + m2*(l * sin(u(3)) * u(4)^2 + g * sin(u(3)) * cos(u(3))) - (f_1k*u(2) + f_1s*m1*g*sgn(u(2))) + 1 / l * cos(u(3))*(f_2k*u(4) + M_sp*sgn(u(4))) )
  "pendulum " : Fcn  Expr=1/(l*(m1 + m2*sin(u(3))^2)) * (-(m1 + m2)* g * sin(u(3)) - u(5)*cos(u(3)) - m2*l*sin(u(3))*cos(u(3))*u(4)^2 + cos(u(3))*(f_1k*u(2) + f_1s*m1*g*sgn(u(2))) - (1 + m1/m2)*(1/l * (f_2k*u(4)+M_sp*sgn(u(4)))))
  rad to degree : Gain  Gain=180/pi
  cart position : Outport
  "pendulum position " : Outport  Port=2
  wires:
  cart/1 -> Integrator3/1  "ddx1"
  Mux2/1 -> "pendulum "/1
  "pendulum "/1 -> Integrator5/1  "ddtheta"
  Integrator5/1 -> Integrator12/1, Mux1/4, Mux2/4  "dtheta"
  Integrator3/1 -> Integrator4/1, Mux2/2, Mux1/2  "dx1"
  Integrator12/1 -> rad to degree/1, Mux1/3, Mux2/3  "theta"
  Mux1/1 -> cart/1
  rad to degree/1 -> "pendulum position "/1
  Integrator4/1 -> cart position/1, Mux2/1, Mux1/1
  controll input/1 -> Mux2/5, Mux1/5

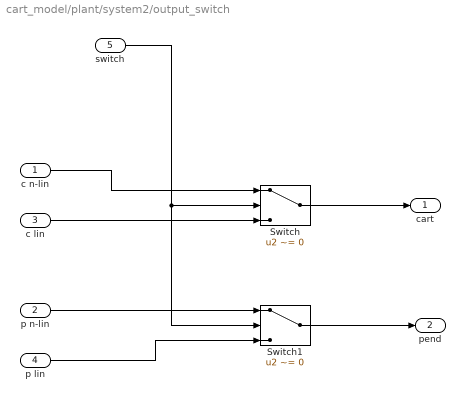
== system cart_model/plant/system2/output_switch ==
  c n-lin : Inport
  p n-lin : Inport  Port=2
  c lin : Inport  Port=3
  p lin : Inport  Port=4
  switch : Inport  Port=5
  Switch : Switch  Criteria=u2 ~= 0  Threshold=1
  Switch1 : Switch  Criteria=u2 ~= 0  Threshold=1
  cart : Outport
  pend : Outport  Port=2
  wires:
  switch/1 -> Switch1/2, Switch/2
  p lin/1 -> Switch1/3
  Switch/1 -> cart/1
  c lin/1 -> Switch/3
  Switch1/1 -> pend/1
  c n-lin/1 -> Switch/1
  p n-lin/1 -> Switch1/1

== matlab function cart_model/Synchronization/MATLAB Function1 ==
  data: u input; y output; m_new input; m_old output
function [y, m_old] = fcn(u, m_new)
%#codegen

threshold = 40;

if(u > 0 && m_new < threshold)
    m_old = m_new + 1;
else
    m_old = m_new;
end

if(m_old == threshold)
    y = 1;
else
    y=0;
end

== matlab function cart_model/MATLAB Function ==
  data: u input; y output; m_new input; m_old output
function [y, m_old] = fcn(u, m_new)
%#codegen

threshold = 40;

if(u > 0 && m_new < threshold)
    m_old = m_new + 1;
else
    m_old = m_new;
end

if(m_old == threshold)
    y = 1;
else
    y=0;
end
